simulink model "DCEE_80400_111_t30s"  (R2024b)
settings: Solver=FixedStepDiscrete  StartTime=0.0  StopTime=3.5  FixedStep=1e-6  RelTol=1e-3
libraries: spsSeriesRLCBranchLib x3, spsStairGeneratorLib x3, spsDiodeLib x2, spsVoltageMeasurementLib x2, spsMosfetLib x1, spsPWMGeneratorDCDCLib x1, spsPVArrayLib x1, spsSeriesRLCLoadLib x1, spspowerguiLib x1
settings Model: Creator=LOUZAZNI  LastModifiedBy=yuyalei
settings SolverCC: AlgebraicLoopSolver=TrustRegion
settings OptimizationCC: ReuseModelBlockBuffer=off
settings DebuggingCC: UnconnectedInputMsg=warning  UnconnectedOutputMsg=warning  UnconnectedLineMsg=warning
settings ModelReferenceCC: EnableRefExpFcnMdlSchedulingChecks=on
settings SFSimCC: CustomCodeUndefinedFunction=UseInterfaceOnly
settings RTWCC: GPUComputeCapability=3.5

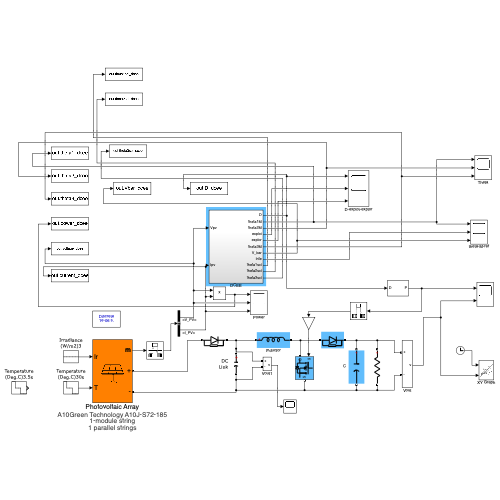
[thumbnail: Simulink's stored preview of the top-level diagram]
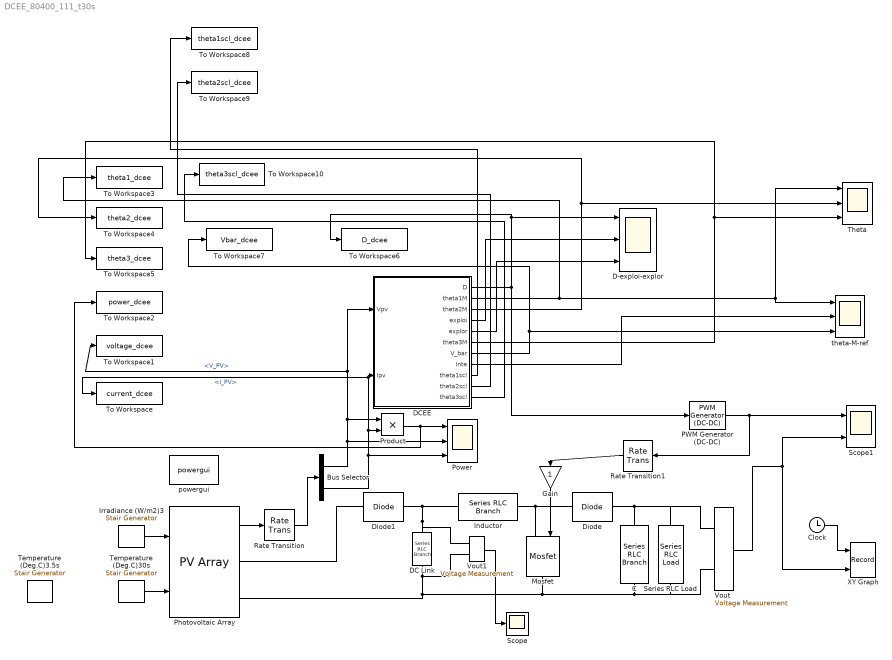
== system DCEE_80400_111_t30s ==
  Bus Selector : BusSelector  OutputSignals=V_PV,I_PV
  C : spsSeriesRLCBranchLib/Series RLC Branch  LConnTagsString=__new0  RConnTagsString=__new0  BranchType=C  Resistance=1  Inductance=1e-3  SetiL0=off  InitialCurrent=0  Capacitance=50e-6  Setx0=off  InitialVoltage=600  Measurements=None
  Clock : Clock
  D-exploi-explor : Scope  NumInputPorts=3
  DC Link : spsSeriesRLCBranchLib/Series RLC Branch  LConnTagsString=__new0  RConnTagsString=__new0  BranchType=C  Resistance=0.001  Inductance=1.0  SetiL0=off  InitialCurrent=0  Capacitance=4000e-6  Setx0=off  InitialVoltage=310  Measurements=None
  DCEE : Subsystem
  Diode : spsDiodeLib/Diode  Ron=0.001  Lon=0  Vf=0.8  IC=0  UseSnubber=off  Rs=500  Cs=250e-9  Measurements=off
  Diode1 : spsDiodeLib/Diode  Ron=0.001  Lon=0  Vf=0.8  IC=0  UseSnubber=off  Rs=500  Cs=250e-9  Measurements=off
  Gain : Gain  OutDataTypeStr=Inherit: Inherit via back propagation
  Inductor : spsSeriesRLCBranchLib/Series RLC Branch  LConnTagsString=__new0  RConnTagsString=__new0  BranchType=L  Resistance=0.01  Inductance=4e-4  SetiL0=off  InitialCurrent=5  Capacitance=1e-6  Setx0=off  InitialVoltage=0  Measurements=None
  Irradiance (W/m2)3 : spsStairGeneratorLib/Stair Generator  t=[0, 0.5, 1, 1.5, 2, 2.5, 3]  e=[1, 1, 1, 1, 1, 1, 1]*1000  Ts=0.0001
  Mosfet : spsMosfetLib/Mosfet  Ron=0.1  Lon=0  Rd=0.01  Vfd=0  IC=0  Rs=1e5  Cs=inf  Measurements=off
  PWM Generator (DC-DC) : spsPWMGeneratorDCDCLib/PWM Generator (DC-DC)  Fsw=10000  Ts=0
  Photovoltaic Array : spsPVArrayLib/PV Array  Npar=1  Nser=1  PlotType=one module @ 25 deg.C & specified irradiances  S_vec=[300]  Temp_C_vec=[ 25 ]  ModuleName=A10Green Technology A10J-S72-185  PlotWhenSelected=off  Pm=184.7016  Ncell=72  Voc=44.14  Isc=5.43  Vm=36.72  Im=5.03  beta_Voc_pc=-0.3616  alpha_Isc_pc=0.041492  beta_Voc=-0.15961  alpha_Isc=0.002253  IL=5.4379  I0=1.8755e-10  nI=0.99182  Rsh=257.1494  Rs=0.37471  RobustModel=off  RobustCellTemperature=313.3991  BAL=on  Tc=1e-6  Tfilter=5e-5
      settings: AttributesFormatString=|
      | %<ModuleName>
      | %<Nser>-module string
      | %<Npar> parallel strings
  Power : Scope  NumInputPorts=3
  Product : Product  RndMeth=Zero
  Rate Transition : RateTransition  OutPortSampleTime=1e-4
  Rate Transition1 : RateTransition  OutPortSampleTime=1e-6
  Scope : Scope
  Scope1 : Scope  NumInputPorts=2
  Series RLC Load : spsSeriesRLCLoadLib/Series RLC Load  LConnTagsString=a  RConnTagsString=__new0  NominalVoltage=30  NominalFrequency=50  ActivePower=50  InductivePower=0  CapacitivePower=0  Setx0=off  InitialVoltage=0  SetiL0=off  InitialCurrent=0  Measurements=None  LoadType=constant Z
  Temperature (Deg.C)3.5s : spsStairGeneratorLib/Stair Generator  t=[0, 0.5, 1, 1.5, 2, 2.5, 3]  e=[80, 80, 40, 40, 0, 0, 0]  Ts=0.0001
  Temperature (Deg.C)30s : spsStairGeneratorLib/Stair Generator  t=[0, 5, 10, 15, 20, 25, 30]  e=[80, 80, 40, 40, 0, 0, 0]  Ts=0.0001
  Theta : Scope  NumInputPorts=3
  To Workspace : ToWorkspace  VariableName=current_dcee  SaveFormat=Timeseries  SampleTime=-1
  To Workspace1 : ToWorkspace  VariableName=voltage_dcee  SaveFormat=Timeseries  SampleTime=-1
  To Workspace10 : ToWorkspace  VariableName=theta3scl_dcee  SaveFormat=Timeseries  SampleTime=-1
  To Workspace2 : ToWorkspace  VariableName=power_dcee  SaveFormat=Timeseries  SampleTime=-1
  To Workspace3 : ToWorkspace  VariableName=theta1_dcee  SaveFormat=Timeseries  SampleTime=-1
  To Workspace4 : ToWorkspace  VariableName=theta2_dcee  SaveFormat=Timeseries  SampleTime=-1
  To Workspace5 : ToWorkspace  VariableName=theta3_dcee  SaveFormat=Timeseries  SampleTime=-1
  To Workspace6 : ToWorkspace  VariableName=D_dcee  SaveFormat=Timeseries  SampleTime=-1
  To Workspace7 : ToWorkspace  VariableName=Vbar_dcee  SaveFormat=Timeseries  SampleTime=-1
  To Workspace8 : ToWorkspace  VariableName=theta1scl_dcee  SaveFormat=Timeseries  SampleTime=-1
  To Workspace9 : ToWorkspace  VariableName=theta2scl_dcee  SaveFormat=Timeseries  SampleTime=-1
  Vout : spsVoltageMeasurementLib/Voltage Measurement  PhasorSimulation=off  OutputType=Complex  PSBequivalent=0
  Vout1 : spsVoltageMeasurementLib/Voltage Measurement  PhasorSimulation=off  OutputType=Complex  PSBequivalent=0
  XY Graph : Record  FileSettingsInternal="{\"entries\":[{\"content\":{\"excelSettings\":{\"content\":{},\"type\":\"Streamout.ExcelSettings\"}},\"type\":\"Streamout.FileSettingStorage\",\"uuid\":\"\"}],\"packageUris\":[\"http:\\/\\/schema.mathworks.com\\/mf0\\/streamout_blocks\\/R2020a\"],\"version\":\"1.0\"}"  Layout=[1 1]  SignalsInternal="{\"entries\":[{\"content\":{\"signals\":[{\"content\":{\"blockPath\":[],\"dimensions\":[1],\"domain\":\"\",\"lineColor\":\"#4dbeee\",\"port\":1,\"signalID\":1,\"signalName\":\"Clock\"},\"type\":\"RecordBlkView.Signal\",\"uuid\":\"\"},{\"content\":{\"blockPath\":[],\"dimensions\":[1],\"domain\":\"\",\"lineColor\":\"#a2142f\",\"port\":2,\"signalID\":2,\"signalName\":\"Vout\"},\"type\":\"RecordBlkView.Signal\",\"uuid\":\"\"}]},\"type\":\"RecordBlkView.InputSignals\",\"uuid\":\"\"}],\"packageUris\":[\"http:\\/\\/schema.mathworks.com\\/mf0\\/streamout_blocks\\/R2020a\"],\"version\":\"1.0\"}"  VisualizationBindings="{\"xyplotplugin\":{\"info\":[{\"series\":[],\"subplotID\":1}]}}"  CompatibilityTag=XY  st=0.0001
  powergui : spspowerguiLib/powergui  Priority=1  SimulationMode=Discrete  SampleTime=1e-6  frequency=60  Iterations=50  frequencyindice=0  Pbase=100e6  ErrMax=1e-4  UnitsV=kV  UnitsW=MW  buscounter=0  FunctionMessages=off  echomessages=off  EnableUseOfTLC=off  CurrentSourceSwitches=off  DisableSnubberDevices=off  DisableRonSwitches=off  DisableVfSwitches=off  DisplayEquations=off  AutomaticDiscreteSolvers=off  SolverType=Tustin/Backward Euler (TBE)  Interpol=off  ExternalGateDelay=off  methode=off  Ts=100  x0status=blocks  SPID=off  SwTol=0  HookPort=off  NonlinearTolerance=0  nMaxIteration=15  ContinueOnMaxIteration=off  RestoreLinks=warning  ResistiveCurrentMeasurement=off  Frange=[0:2:500]  Ylog=off  Xlog=on  ShowGrid=off  save=off  variable=ZData  structure=0  ZoomFFT=off  StartTime=0.0  cycles=1  DisplayStyle=1  fundamental=60  FreqAxis=off  MaxFrequency=1000  frequencyindicesteady=1  RmsSteady=1  display=off
  theta-M-ref : Scope  NumInputPorts=3
  wires:
  Vout1/1 -> Scope/1
  Vout/1 -> XY Graph/2, Scope1/2
  Clock/1 -> XY Graph/1
  Bus Selector/1 -> To Workspace1/1, DCEE/1(Vpv), Product/1, Power/2  "<V_PV>"
  Photovoltaic Array/1 -> Rate Transition/1
  PWM Generator (DC-DC)/1 -> Scope1/1, Rate Transition1/1
  Bus Selector/2 -> DCEE/2(Ipv), To Workspace/1, Product/2, Power/3  "<I_PV>"
  Irradiance (W/m2)3/1 -> Photovoltaic Array/1
  Temperature (Deg.C)30s/1 -> Photovoltaic Array/2
  Product/1 -> Power/1, To Workspace2/1
  Gain/1 -> Mosfet/1
  DCEE/4(exploi) -> D-exploi-explor/2
  DCEE/5(explor) -> D-exploi-explor/3
  DCEE/7(V_bar) -> To Workspace7/1, theta-M-ref/3
  DCEE/3(theta2M) -> To Workspace4/1, Theta/2
  DCEE/1(D) -> PWM Generator (DC-DC)/1, D-exploi-explor/1, To Workspace6/1
  Rate Transition/1 -> Bus Selector/1
  Rate Transition1/1 -> Gain/1
  DCEE/2(theta1M) -> To Workspace3/1, Theta/1, theta-M-ref/1
  DCEE/6(theta3M) -> To Workspace5/1, Theta/3
  DCEE/8(Inte) -> theta-M-ref/2
  DCEE/9(theta1scl) -> To Workspace8/1
  DCEE/10(theta2scl) -> To Workspace9/1
  DCEE/11(theta3scl) -> To Workspace10/1
  connections:
  Photovoltaic Array/RConn2 -- Vout1/LConn2 -- DC Link/RConn1 -- Mosfet/RConn1 -- Vout/LConn2 -- Series RLC Load/RConn1 -- C/RConn1
  Mosfet/LConn1 -- Inductor/RConn1 -- Diode/LConn1
  Diode1/RConn1 -- Vout1/LConn1 -- DC Link/LConn1 -- Inductor/LConn1
  C/LConn1 -- Diode/RConn1 -- Vout/LConn1 -- Series RLC Load/LConn1
  Photovoltaic Array/RConn1 -- Diode1/LConn1

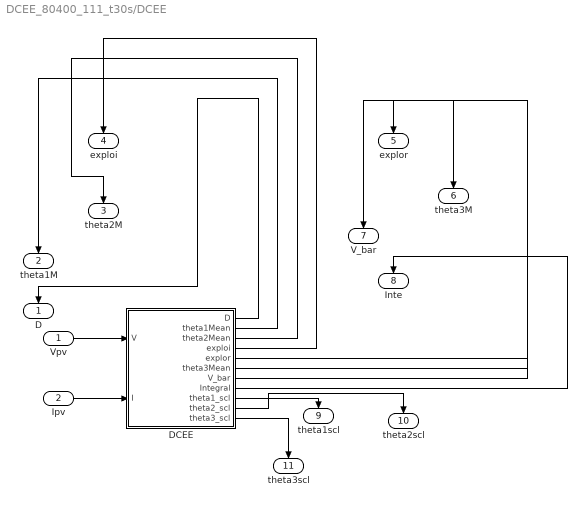
== system DCEE_80400_111_t30s/DCEE ==
  Vpv : Inport
  Ipv : Inport  Port=2
  DCEE : MATLAB Function  TreatAsAtomicUnit=on
  D : Outport  VectorParamsAs1DForOutWhenUnconnected=off
  theta1M : Outport  Port=2  VectorParamsAs1DForOutWhenUnconnected=off
  theta2M : Outport  Port=3  VectorParamsAs1DForOutWhenUnconnected=off
  exploi : Outport  Port=4  VectorParamsAs1DForOutWhenUnconnected=off
  explor : Outport  Port=5  VectorParamsAs1DForOutWhenUnconnected=off
  theta3M : Outport  Port=6  VectorParamsAs1DForOutWhenUnconnected=off
  V_bar : Outport  Port=7  VectorParamsAs1DForOutWhenUnconnected=off
  Inte : Outport  Port=8  VectorParamsAs1DForOutWhenUnconnected=off
  theta1scl : Outport  Port=9  VectorParamsAs1DForOutWhenUnconnected=off
  theta2scl : Outport  Port=10  VectorParamsAs1DForOutWhenUnconnected=off
  theta3scl : Outport  Port=11  VectorParamsAs1DForOutWhenUnconnected=off
  wires:
  DCEE/1(D) -> D/1
  Vpv/1 -> DCEE/1(V)
  Ipv/1 -> DCEE/2(I)
  DCEE/2(theta1Mean) -> theta1M/1
  DCEE/3(theta2Mean) -> theta2M/1
  DCEE/4(exploi) -> exploi/1
  DCEE/5(explor) -> explor/1
  DCEE/6(theta3Mean) -> theta3M/1
  DCEE/7(V_bar) -> V_bar/1
  DCEE/8(Integral) -> Inte/1
  DCEE/9(theta1_scl) -> theta1scl/1
  DCEE/10(theta2_scl) -> theta2scl/1
  DCEE/11(theta3_scl) -> theta3scl/1

== matlab function DCEE_80400_111_t30s/DCEE/DCEE ==
  data: D output; V input; I input; theta1Mean output; theta2Mean output; exploi output; explor output; theta3Mean output; V_bar output; Integral output; theta1_scl output; theta2_scl output; theta3_scl output
                               
function [D, theta1Mean, theta2Mean, exploi, explor, theta3Mean, V_bar, Integral, ...
          theta1_scl, theta2_scl, theta3_scl] = DCEE(V, I)
    
    % Dinit = 0.01;  
    Dmax = 1 ;
    Dmin = 0.001;
    
    thetamin1 = 0.01;
    thetamax1 = 1;
    thetamin2 = 9;
    thetamax2 = 12;
    thetamin3 = 24;
    thetamax3 = 26; 

    D = 0; 
    N = 2;
    % N = 20; 
    tau_d = 2000;  % 2000 = 5 × 400: sample every 5th point, up to 400 data points
    tau = 0.001;

    %%
    persistent Vold  M theta Int   ...
               V_store Reward_store Jbelief_store  ...
               theta1_sum_cl_store theta2_sum_cl_store theta3_sum_cl_store ...
    
    dataType = 'double';
    if isempty(Vold)
        Vold=0;
        M=1;
        V = 0;
        Int = 0;
    
        theta1 = thetamin1 + (thetamax1 - thetamin1)*rand(N,1);
        theta2 = thetamin2 + (thetamax2 - thetamin2)*rand(N,1);
        theta3 = thetamin3 + (thetamax3 - thetamin3)*rand(N,1); 
    
        theta = [theta1 theta2 theta3];

        V_store = zeros(tau_d,1);
        Reward_store = zeros(tau_d,1);

        Jbelief_store = zeros(tau_d, N);

        theta1_sum_cl_store = zeros(tau_d, N);
        theta2_sum_cl_store = zeros(tau_d, N);
        theta3_sum_cl_store = zeros(tau_d, N);
    end

    numl1 = [M tau_d];
    numl = min(numl1);

    %% design parameters
    Ts = 1e-04;
    
    delta_expoi = 0.18; 
    delta_expor = 0.1;
    ki = 10; 

    eta1 = 0.0005;
    eta2 = 0.5;
    eta3 = 0.001;
    eta = [eta1; eta2; eta3];

    Numl2 = 1.5/Ts;
    Numl3 = 2.5/Ts;
    Numl4 = 3.5/Ts;
  
    %% parameter estimation
    RewardSim = V*I;
    noise = 0.5*randn(size(RewardSim));
    RewardSim = RewardSim + noise;
    
    Reward_new = RewardSim;
    
    Jbelief = reward(theta, V);
    Jbelief_new = Jbelief;

    Jbelief_store = cat(1, Jbelief_store(2:end,:), Jbelief_new');
   
    theta1 = theta(:,1);
    theta2 = theta(:,2);
    theta3 = theta(:,3); 
    
    %% concurrent learning
    V_new = V;

    %%
    dd = 5;
    V_store = cat(1, V_store(2:end), V_new);
    Reward_store = cat(1, Reward_store(2:end), Reward_new);
 
    for j = 1:tau_d
        theta1_sum_cl = (reward(theta, V_store(j)) - Reward_store(j)*ones(N,1)).*(-V_store(j).^2);
        theta2_sum_cl = (reward(theta, V_store(j)) - Reward_store(j)*ones(N,1)).*V_store(j);
        theta3_sum_cl = (reward(theta, V_store(j)) - Reward_store(j)*ones(N,1)).*(-1);
        theta1_sum_cl_new = theta1_sum_cl;
        theta2_sum_cl_new = theta2_sum_cl;
        theta3_sum_cl_new = theta3_sum_cl;
        
        if mod(j,dd)==0
        theta1_sum_cl_store = cat(1, theta1_sum_cl_store(2:end,:), theta1_sum_cl_new');
        theta2_sum_cl_store = cat(1, theta2_sum_cl_store(2:end,:), theta2_sum_cl_new');
        theta3_sum_cl_store = cat(1, theta3_sum_cl_store(2:end,:), theta3_sum_cl_new');
        elseif j==1
        theta1_sum_cl_store = cat(1, theta1_sum_cl_store(2:end,:), theta1_sum_cl_new');
        theta2_sum_cl_store = cat(1, theta2_sum_cl_store(2:end,:), theta2_sum_cl_new');
        theta3_sum_cl_store = cat(1, theta3_sum_cl_store(2:end,:), theta3_sum_cl_new');  
        end
        
    end
    
    if  tau_d == 0
        theta1 = theta1 - eta1.*(Jbelief - RewardSim*ones(N,1)).*(-V.^2)*Ts./(1+V.^4*eta1);
        theta2 = theta2 - eta2.*(Jbelief - RewardSim*ones(N,1)).*V*Ts./(1+V.^2*eta2);
        theta3 = theta3 - eta3.*(Jbelief - RewardSim*ones(N,1)).*(-1)*Ts./(1+1*eta3);
    else
        theta1_sum_cl = sum(theta1_sum_cl_store', 2);
        theta2_sum_cl = sum(theta2_sum_cl_store', 2);
        theta3_sum_cl = sum(theta3_sum_cl_store', 2);
    
        theta1 = theta1 - eta1.*theta1_sum_cl*Ts/(1+V.^4*eta1);
        theta2 = theta2 - eta2.*theta2_sum_cl*Ts/(1+V.^2*eta2);
        theta3 = theta3 - eta3.*theta3_sum_cl*Ts/(1+1*eta3);
    end
    
    %% boundary of parameters
    theta = [theta1 theta2 theta3];
        
    theta1Mean = mean(theta1);
    theta2Mean = mean(theta2);
    theta3Mean = mean(theta3);
      
    %% dual controller
    [future_mean, future_variance] = predicted_mean_variance(theta, V, eta);
    
    V_bar = future_mean(2)/(2*future_mean(1));
    
    exploitation_gradient = (V - V_bar);
   
    D_sat = max(min(D, Dmax), Dmin); 
    
    Integral = Int + (ki*exploitation_gradient + (D - D_sat)/tau)*Ts;

    exploration_gradient = (get_variance_gradient(theta, V, eta));
    
    dual =  delta_expoi*exploitation_gradient + delta_expor*exploration_gradient;
    
    D = dual;
     
    %% outputs 
    if D >= Dmax
        D = Dmax;
    elseif D <= Dmin
        D = Dmin;
    else D = D;
    end
    
    M = M + 1;
    Int = Integral; 
  
    exploi = exploitation_gradient;
    explor = exploration_gradient; 
    
    theta1_scl = theta1_sum_cl;
    theta2_scl = theta2_sum_cl;
    theta3_scl = theta3_sum_cl;

    %% Functions
    %% function: reward
        function [ J ] = reward(theta, y)
    
            theta11 = theta(:,1);
            theta12 = theta(:,2);
            theta13 = theta(:,3); 
  
            J = -theta11.*y^2 + theta12.*y - theta13;
        end
    
    %% function: predicted_mean_variance
        function [future_mean, future_variance] = predicted_mean_variance(theta, x, eta)
    
            [GradFa] = gradientF(theta, x);
             
            eta1 = eta(1); eta2 = eta(2); eta3 = eta(3);
    
            future_thetaA1 = theta(:,1) - eta1.*GradFa.*(-x.^2)*Ts./(1+x.^4*eta1);
            future_thetaA2 = theta(:,2) - eta2.*GradFa.*(x)*Ts./(1+x.^2*eta2);
            future_thetaA3 = theta(:,3) - eta3.*GradFa.*(-1)*Ts./(1+eta3);

            future_thetaA = [future_thetaA1 future_thetaA2 future_thetaA3];
            
            future_mean = [mean(future_thetaA1) mean(future_thetaA2) mean(future_thetaA3)]; 
    
            future_variance = var(future_thetaA);
        end
    
    %% function: gradientF
        function [GradFa] = gradientF(theta, x)
            currentMean = mean(theta);
    
            predictedJ = reward(currentMean, x);  % predicted mean of future reward based on current belief
    
            individualJ = reward(theta, x);
    
            GradFa = (individualJ - predictedJ);
        end
    
    %% function: get_variance_gradient
        function [variance_gradient] = get_variance_gradient(theta, x, eta)
            delta_x = 1e-4;
            % delta_x denotes the size of step
            [GradFa] = gradientF(theta, x);
            eta1 = eta(1); eta2 = eta(2); eta3 = eta(3);
            
            future_thetaA1 = theta(:,1) - eta1.*GradFa.*(-x.^2)*Ts./(1+x.^4*eta1);
            future_thetaA2 = theta(:,2) - eta2.*GradFa.*(x)*Ts./(1+x.^2*eta2);
            future_thetaA3 = theta(:,3) - eta3.*GradFa.*(-1)*Ts./(1+eta3);

            future_thetaA = [future_thetaA1 future_thetaA2 future_thetaA3];
            future_mean = [mean(future_thetaA1) mean(future_thetaA2) mean(future_thetaA3)];
            future_variance = var(future_thetaA) ;
   
            [GradFa_delta] = gradientF(theta, x+delta_x);
    
            future_thetaA1_delta = theta(:,1) - eta1.*GradFa_delta.*(-x.^2)*Ts./(1+x.^4*eta1);
            future_thetaA2_delta = theta(:,2) - eta2.*GradFa_delta.*(x)*Ts./(1+x.^2*eta2);
            future_thetaA3_delta = theta(:,3) - eta3.*GradFa_delta.*(-1)*Ts./(1+eta3);

            future_thetaA_delta = [future_thetaA1_delta future_thetaA2_delta future_thetaA3_delta];
            future_mean = [mean(future_thetaA1_delta) mean(future_thetaA2_delta) mean(future_thetaA3_delta)];

            future_variance_delta = var(future_thetaA_delta) ;
    
            variance_gradient1 = (future_variance_delta-future_variance)./delta_x;
            variance_gradient = sum(variance_gradient1);
        end
   
    end
